simulink model "firstsimulink"  (R2021a)
settings: Solver=VariableStepAuto  StartTime=0.0  StopTime=10.0  RelTol=1e-3
settings Model: Creator=arnav  LastModifiedBy=arnav

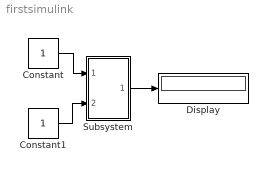
== system firstsimulink ==
  Constant : Constant
  Constant1 : Constant
  Display : Display
  Subsystem : Subsystem
  wires:
  Constant/1 -> Subsystem/1(In1)
  Constant1/1 -> Subsystem/2(In2)
  Subsystem/1(Out1) -> Display/1

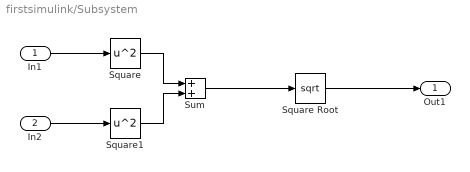
== system firstsimulink/Subsystem ==
  In1 : Inport
  In2 : Inport  Port=2
  Square : Math  Operator=square  SaturateOnIntegerOverflow=on
  Square Root : Sqrt  SaturateOnIntegerOverflow=on
  Square1 : Math  Operator=square  SaturateOnIntegerOverflow=on
  Sum : Sum  Inputs=+|+
  Out1 : Outport
  wires:
  In1/1 -> Square/1
  Sum/1 -> Square Root/1
  In2/1 -> Square1/1
  Square1/1 -> Sum/2
  Square/1 -> Sum/1
  Square Root/1 -> Out1/1
